simulink model "filter_mech_ell_noise"  (R2025b)
settings: Solver=VariableStepAuto  StartTime=0.0  StopTime=time(end)  RelTol=1e-3
values from neighbouring files (symbols this model uses):
  rpy = zeros(length(time),3)    [test_traj_gen_v2 1.m]    (also in test_traj_gen_v2.m)
  ST = 1/100    (= 0.01)    [test_traj_gen_v2 1.m]    (also in test_traj_gen_v2.m)
  vel_n = vel_n_f    [test_traj_gen_v2 1.m]    (also in test_traj_gen_v2.m)
undefined symbols (not defined in the file or in its folder): DiscIntNeverNeededParam
settings Model: Creator=Lorenzo  LastModifiedBy=roly2
settings RTWCC: GPUComputeCapability=3.5

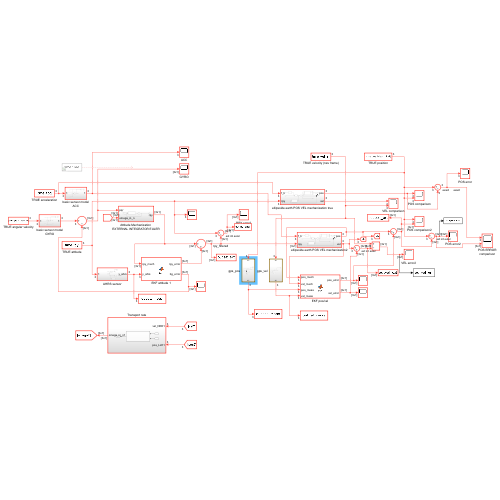
[thumbnail: Simulink's stored preview of the top-level diagram]
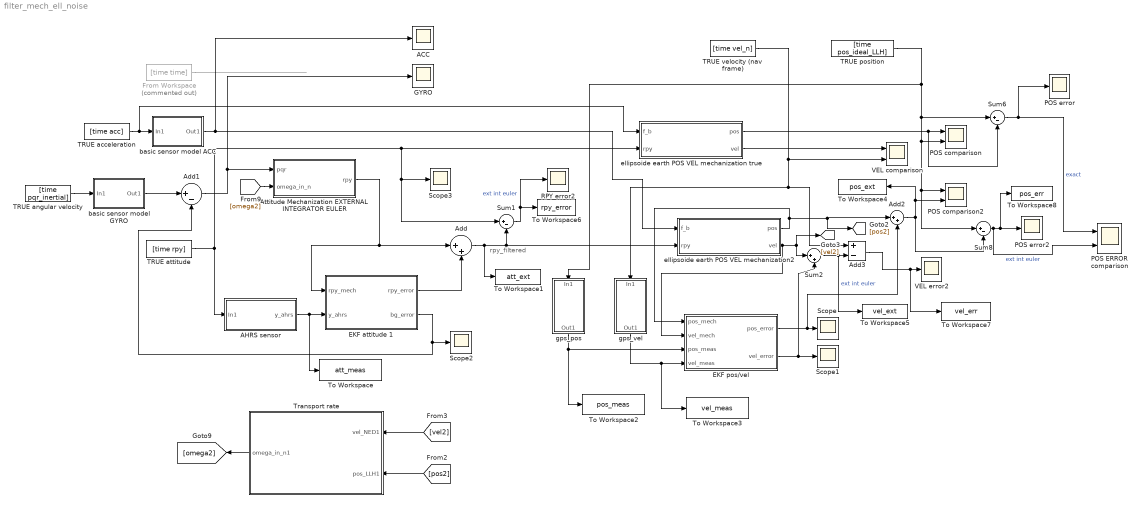
== system filter_mech_ell_noise ==
  note: rpy_filtered
  ACC : Scope
      settings: ActiveDisplayYMinimum=-11.440992557737301  ActiveDisplayYMaximum=2.4820081212415044  DataLoggingVariableName=ScopeData5
  AHRS sensor : Subsystem
  Add : Sum  Inputs=|++
  Add1 : Sum  Inputs=|+-
  Add2 : Sum  Inputs=|++
  Add3 : Sum  Inputs=+-
  Attitude Mechanization EXTERNAL INTEGRATOR EULER : Subsystem
  EKF attitude 1 : MATLAB Function  TreatAsAtomicUnit=on
  EKF pos/vel : MATLAB Function  TreatAsAtomicUnit=on
  From Workspace : FromWorkspace  Commented=on  VariableName=[time time]  SampleTime=ST
  GYRO : Scope
      settings: ActiveDisplayYMinimum=-0.0020882472519492545  ActiveDisplayYMaximum=0.00068115329120505431  DataLoggingVariableName=ScopeData12
  POS ERROR comparison : Scope  NumInputPorts=2
      settings: ActiveDisplayYMinimum=-0.463446142414341  ActiveDisplayYMaximum=0.1393650133582014  DataLoggingVariableName=ScopeData11
  POS comparison : Scope  NumInputPorts=2
      settings: ActiveDisplayYMinimum=19774.997277480568  ActiveDisplayYMaximum=20025.000302502158  DataLoggingVariableName=ScopeData2
  POS comparison2 : Scope  NumInputPorts=2
      settings: ActiveDisplayYMinimum=19774.812142318573  ActiveDisplayYMaximum=20025.022393794803
  POS error : Scope
      settings: ActiveDisplayYMinimum=-0.00026486838760320092  ActiveDisplayYMaximum=0.0023749580650473945  DataLoggingVariableName=ScopeData6
  POS error2 : Scope
      settings: ActiveDisplayYMinimum=-0.507273817207988  ActiveDisplayYMaximum=0.53432806462160443  DataLoggingVariableName=ScopeData8
  RPY error2 : Scope
      settings: ActiveDisplayYMinimum=-0.02159298222479724  ActiveDisplayYMaximum=0.026097778303773897
  Scope{,1..3} (4 alike) : Scope
      Scope settings: ActiveDisplayYMinimum=-5.2228791618423713  ActiveDisplayYMaximum=15.526847222191225
      Scope1 settings: ActiveDisplayYMinimum=0.5852793052063231  ActiveDisplayYMaximum=0.6306251008108662  DataLoggingVariableName=ScopeData9
      Scope2 settings: ActiveDisplayYMinimum=-0.0046074754298184107  ActiveDisplayYMaximum=0.0078155605686823729  DataLoggingVariableName=ScopeData16
      Scope3 settings: DataLoggingVariableName=ScopeData17
  Sum1 : Sum  Inputs=|+-
  Sum2 : Sum  Inputs=|++
  Sum6 : Sum  Inputs=|+-
  Sum8 : Sum  Inputs=|+-
  TRUE acceleration : FromWorkspace  VariableName=[time acc]  SampleTime=ST
  TRUE angular velocity : FromWorkspace  VariableName=[time pqr_inertial]  SampleTime=ST
  TRUE attitude : FromWorkspace  VariableName=[time rpy]  SampleTime=ST
  TRUE position : FromWorkspace  VariableName=[time pos_ideal_LLH]  SampleTime=ST
  TRUE velocity (nav frame) : FromWorkspace  VariableName=[time vel_n]  SampleTime=ST
  To Workspace : ToWorkspace  VariableName=att_meas  SaveFormat=Timeseries  SampleTime=-1
  To Workspace1 : ToWorkspace  VariableName=att_ext  SaveFormat=Timeseries  SampleTime=-1
  To Workspace2 : ToWorkspace  VariableName=pos_meas  SaveFormat=Timeseries  SampleTime=-1
  To Workspace3 : ToWorkspace  VariableName=vel_meas  SaveFormat=Timeseries  SampleTime=-1
  To Workspace4 : ToWorkspace  VariableName=pos_ext  SaveFormat=Timeseries  SampleTime=-1
  To Workspace5 : ToWorkspace  VariableName=vel_ext  SaveFormat=Timeseries  SampleTime=-1
  To Workspace6 : ToWorkspace  VariableName=rpy_error  SaveFormat=Timeseries  SampleTime=-1
  To Workspace7 : ToWorkspace  VariableName=vel_err  SaveFormat=Timeseries  SampleTime=-1
  To Workspace8 : ToWorkspace  VariableName=pos_err  SaveFormat=Timeseries  SampleTime=-1
  Transport rate : Subsystem
  VEL comparison : Scope  NumInputPorts=2
      settings: ActiveDisplayYMinimum=-163.77870347813263  ActiveDisplayYMaximum=201.30598005002113  DataLoggingVariableName=ScopeData3
  VEL error2 : Scope
      settings: ActiveDisplayYMinimum=-0.087937577094350031  ActiveDisplayYMaximum=0.084021536567730273  DataLoggingVariableName=ScopeData4
  basic sensor model ACC : Subsystem
  basic sensor model GYRO : Subsystem
  ellipsoide earth POS VEL mechanization true : Subsystem
  ellipsoide earth POS VEL mechanization2 : Subsystem
  gps_pos : Subsystem
  gps_vel : Subsystem
  wires:
  From Workspace/1 -> ?
  TRUE position/1 -> gps_pos/1(In1), POS comparison/2, Sum8/1, POS comparison2/1, Sum6/1
  TRUE velocity (nav frame)/1 -> Add3/1, gps_vel/1(In1), VEL comparison/2
  ellipsoide earth POS VEL mechanization true/1(pos) -> Sum6/2, POS comparison/1
  ellipsoide earth POS VEL mechanization true/2(vel) -> VEL comparison/1
  TRUE angular velocity/1 -> basic sensor model GYRO/1(In1)
  Attitude Mechanization EXTERNAL INTEGRATOR EULER/1(rpy) -> EKF attitude 1/1(rpy_mech), Add/1
  Sum1/1 -> To Workspace6/1, RPY error2/1  "ext int euler"
  TRUE attitude/1 -> AHRS sensor/1(In1), Scope3/1, Sum1/1, ellipsoide earth POS VEL mechanization true/2(rpy)
  Sum6/1 -> POS ERROR comparison/1, POS error/1  "exact"
  Sum8/1 -> POS ERROR comparison/2, To Workspace8/1, POS error2/1  "ext int euler"
  ellipsoide earth POS VEL mechanization2/1(pos) -> EKF pos/vel/1(pos_mech), [pos2], Add2/1
  basic sensor model ACC/1(Out1) -> ACC/1, ellipsoide earth POS VEL mechanization2/1(f_b)
  TRUE acceleration/1 -> ellipsoide earth POS VEL mechanization true/1(f_b), basic sensor model ACC/1(In1)
  basic sensor model GYRO/1(Out1) -> Add1/1
  ellipsoide earth POS VEL mechanization2/2(vel) -> EKF pos/vel/2(vel_mech), Sum2/1, [vel2]
  [omega2] -> Attitude Mechanization EXTERNAL INTEGRATOR EULER/2(omega_in_n)
  [vel2] -> Transport rate/1(vel_NED1)
  [pos2] -> Transport rate/2(pos_LLH1)
  Transport rate/1(omega_in_n1) -> [omega2]
  EKF attitude 1/2(bg_error) -> Scope2/1, Add1/2
  AHRS sensor/1(y_ahrs) -> To Workspace/1, EKF attitude 1/2(y_ahrs)
  EKF attitude 1/1(rpy_error) -> Add/2
  Add/1 -> To Workspace1/1, Sum1/2, ellipsoide earth POS VEL mechanization2/2(rpy)
  Add1/1 -> Attitude Mechanization EXTERNAL INTEGRATOR EULER/1(pqr), GYRO/1
  EKF pos/vel/2(vel_error) -> Scope1/1, Sum2/2
  EKF pos/vel/1(pos_error) -> Add2/2, Scope/1
  Add2/1 -> POS comparison2/2, To Workspace4/1, Sum8/2
  gps_pos/1(Out1) -> To Workspace2/1, EKF pos/vel/3(pos_meas)
  gps_vel/1(Out1) -> To Workspace3/1, EKF pos/vel/4(vel_meas)
  Sum2/1 -> To Workspace5/1, Add3/2  "ext int euler"
  Add3/1 -> To Workspace7/1, VEL error2/1

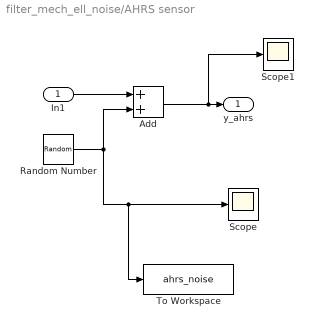
== system filter_mech_ell_noise/AHRS sensor ==
  In1 : Inport
  Add : Sum
  Random Number : RandomNumber  Mean=[0 0 0]  Variance=[0.0003 0.0003 0.0012]  Seed=[6 7 8]  SampleTime=ST
  Scope : Scope
      settings: ActiveDisplayYMinimum=-0.227023215913163  ActiveDisplayYMaximum=0.20537169700863794  DataLoggingVariableName=ScopeData13
  Scope1 : Scope
      settings: ActiveDisplayYMinimum=-0.036488467831931028  ActiveDisplayYMaximum=0.035623775404670058  DataLoggingVariableName=ScopeData14
  To Workspace : ToWorkspace  VariableName=ahrs_noise  SaveFormat=Timeseries  SampleTime=-1
  y_ahrs : Outport
  wires:
  Add/1 -> Scope1/1, y_ahrs/1
  In1/1 -> Add/1
  Random Number/1 -> To Workspace/1, Scope/1, Add/2

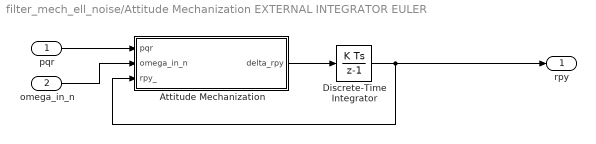
== system filter_mech_ell_noise/Attitude Mechanization EXTERNAL INTEGRATOR EULER ==
  pqr : Inport
  omega_in_n : Inport  Port=2
  Attitude Mechanization : MATLAB Function  TreatAsAtomicUnit=on
  Discrete-Time Integrator : DiscreteIntegrator  InitialCondition=rpy(1,:)'  SampleTime=ST  ICPrevOutput=DiscIntNeverNeededParam  ICPrevScaledInput=DiscIntNeverNeededParam
  rpy : Outport
  wires:
  Discrete-Time Integrator/1 -> rpy/1, Attitude Mechanization/3(rpy_)
  pqr/1 -> Attitude Mechanization/1(pqr)
  Attitude Mechanization/1(delta_rpy) -> Discrete-Time Integrator/1
  omega_in_n/1 -> Attitude Mechanization/2(omega_in_n)

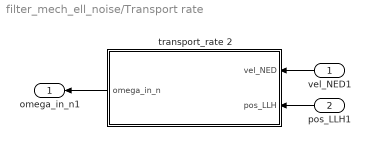
== system filter_mech_ell_noise/Transport rate ==
  vel_NED1 : Inport
  pos_LLH1 : Inport  Port=2
  transport_rate 2 : MATLAB Function  TreatAsAtomicUnit=on
  omega_in_n1 : Outport
  wires:
  pos_LLH1/1 -> transport_rate 2/2(pos_LLH)
  transport_rate 2/1(omega_in_n) -> omega_in_n1/1
  vel_NED1/1 -> transport_rate 2/1(vel_NED)

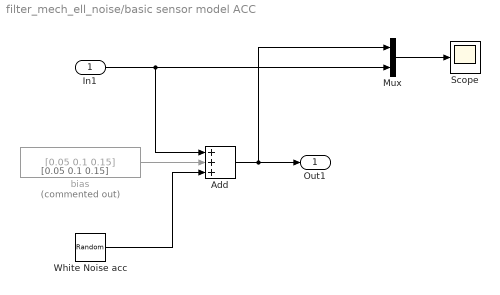
== system filter_mech_ell_noise/basic sensor model ACC ==
  note: [0.05 0.1 0.15]
  In1 : Inport
  Add : Sum  Inputs=+++
  Mux : Mux  Inputs=2
  Scope : Scope
      settings: ActiveDisplayYMinimum=-0.7520653966044506  ActiveDisplayYMaximum=0.75172983316287767
  White Noise acc : RandomNumber  DisableCoverage=on  Mean=[0 0 0 ]  Variance=[0.05 0.05 0.05].^2  Seed=[1 2 3]  SampleTime=ST
  bias : Constant  Commented=on  Value=[0.05 0.1 0.15]
  Out1 : Outport
  wires:
  In1/1 -> Mux/2, Add/1
  White Noise acc/1 -> Add/3
  bias/1 -> Add/2
  Mux/1 -> Scope/1
  Add/1 -> Mux/1, Out1/1

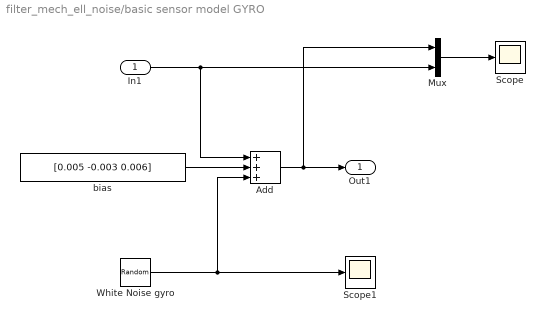
== system filter_mech_ell_noise/basic sensor model GYRO ==
  In1 : Inport
  Add : Sum  Inputs=+++
  Mux : Mux  Inputs=2
  Scope : Scope
      settings: ActiveDisplayYMinimum=-0.018561300716746276  ActiveDisplayYMaximum=0.027069948726320941  DataLoggingVariableName=ScopeData2
  Scope1 : Scope
      settings: ActiveDisplayYMinimum=-1  ActiveDisplayYMaximum=1  DataLoggingVariableName=ScopeData7
  White Noise gyro : RandomNumber  DisableCoverage=on  Mean=[0 0 0]  Variance=[0.003 0.003 0.003].^2  Seed=[4 5 6]  SampleTime=ST
  bias : Constant  Value=[0.005 -0.003 0.006]
  Out1 : Outport
  wires:
  White Noise gyro/1 -> Scope1/1, Add/3
  bias/1 -> Add/2
  Mux/1 -> Scope/1
  In1/1 -> Mux/2, Add/1
  Add/1 -> Mux/1, Out1/1

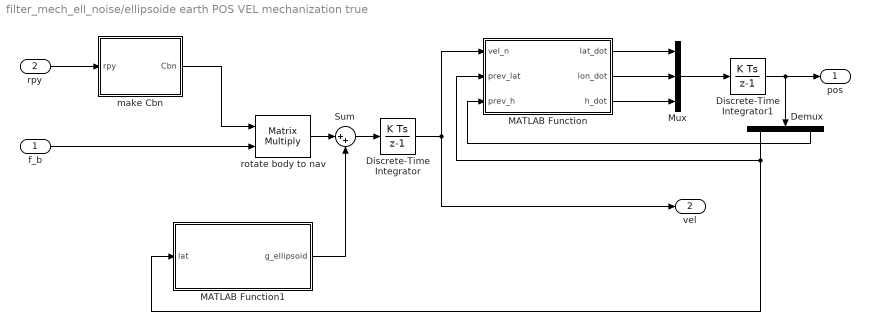
== system filter_mech_ell_noise/ellipsoide earth POS VEL mechanization true ==
  f_b : Inport
  rpy : Inport  Port=2
  Demux : Demux  Outputs=3
  Discrete-Time Integrator : DiscreteIntegrator  InitialCondition=vel_n(1,:)  SampleTime=-1  ICPrevOutput=DiscIntNeverNeededParam  ICPrevScaledInput=DiscIntNeverNeededParam
  Discrete-Time Integrator1 : DiscreteIntegrator  InitialCondition=[40.8522 * pi/180 ; 14.2681 * pi/180 ; 20000]  SampleTime=-1  ICPrevOutput=DiscIntNeverNeededParam  ICPrevScaledInput=DiscIntNeverNeededParam
  MATLAB Function : MATLAB Function  TreatAsAtomicUnit=on
  MATLAB Function1 : MATLAB Function  TreatAsAtomicUnit=on
  Mux : Mux  Inputs=3
  Sum : Sum  Inputs=|++
  make Cbn : MATLAB Function  TreatAsAtomicUnit=on
  rotate body to nav : Product  Multiplication=Matrix(*)
  pos : Outport
  vel : Outport  Port=2
  wires:
  rotate body to nav/1 -> Sum/1
  MATLAB Function1/1(g_ellipsoid) -> Sum/2
  Discrete-Time Integrator/1 -> MATLAB Function/1(vel_n), vel/1
  make Cbn/1(Cbn) -> rotate body to nav/1
  Sum/1 -> Discrete-Time Integrator/1
  f_b/1 -> rotate body to nav/2
  rpy/1 -> make Cbn/1(rpy)
  MATLAB Function/3(h_dot) -> Mux/3
  MATLAB Function/2(lon_dot) -> Mux/2
  MATLAB Function/1(lat_dot) -> Mux/1
  Mux/1 -> Discrete-Time Integrator1/1
  Discrete-Time Integrator1/1 -> pos/1, Demux/1
  Demux/1 -> MATLAB Function1/1(lat), MATLAB Function/2(prev_lat)
  Demux/3 -> MATLAB Function/3(prev_h)

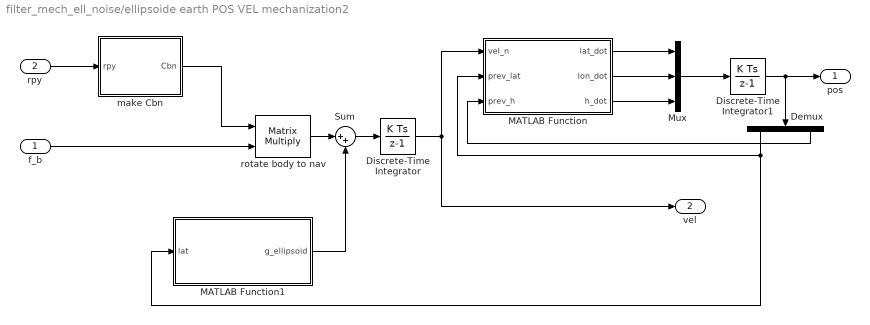
== system filter_mech_ell_noise/ellipsoide earth POS VEL mechanization2 ==
  f_b : Inport
  rpy : Inport  Port=2
  Demux : Demux  Outputs=3
  Discrete-Time Integrator : DiscreteIntegrator  InitialCondition=vel_n(1,:)  SampleTime=-1  ICPrevOutput=DiscIntNeverNeededParam  ICPrevScaledInput=DiscIntNeverNeededParam
  Discrete-Time Integrator1 : DiscreteIntegrator  InitialCondition=[40.8522 * pi/180 ; 14.2681 * pi/180 ; 20000]  SampleTime=-1  ICPrevOutput=DiscIntNeverNeededParam  ICPrevScaledInput=DiscIntNeverNeededParam
  MATLAB Function : MATLAB Function  TreatAsAtomicUnit=on
  MATLAB Function1 : MATLAB Function  TreatAsAtomicUnit=on
  Mux : Mux  Inputs=3
  Sum : Sum  Inputs=|++
  make Cbn : MATLAB Function  TreatAsAtomicUnit=on
  rotate body to nav : Product  Multiplication=Matrix(*)
  pos : Outport
  vel : Outport  Port=2
  wires:
  rotate body to nav/1 -> Sum/1
  Discrete-Time Integrator/1 -> MATLAB Function/1(vel_n), vel/1
  make Cbn/1(Cbn) -> rotate body to nav/1
  Sum/1 -> Discrete-Time Integrator/1
  f_b/1 -> rotate body to nav/2
  rpy/1 -> make Cbn/1(rpy)
  MATLAB Function/3(h_dot) -> Mux/3
  MATLAB Function/2(lon_dot) -> Mux/2
  MATLAB Function/1(lat_dot) -> Mux/1
  Mux/1 -> Discrete-Time Integrator1/1
  Discrete-Time Integrator1/1 -> pos/1, Demux/1
  Demux/3 -> MATLAB Function/3(prev_h)
  Demux/1 -> MATLAB Function1/1(lat), MATLAB Function/2(prev_lat)
  MATLAB Function1/1(g_ellipsoid) -> Sum/2

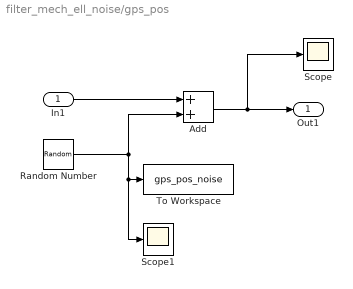
== system filter_mech_ell_noise/gps_pos ==
  In1 : Inport
  Add : Sum
  Random Number : RandomNumber  Mean=[0 0 0]  Variance=[1.5364e-13 1.5364e-13 12.25]  Seed=[3 4 5]  SampleTime=0.1
  Scope : Scope
      settings: ActiveDisplayYMinimum=20000.673472160557  ActiveDisplayYMaximum=20007.042526358724  DataLoggingVariableName=ScopeData15
  Scope1 : Scope
      settings: DataLoggingVariableName=ScopeData18
  To Workspace : ToWorkspace  VariableName=gps_pos_noise  SaveFormat=Timeseries  SampleTime=-1
  Out1 : Outport
  wires:
  Random Number/1 -> Scope1/1, To Workspace/1, Add/2
  Add/1 -> Scope/1, Out1/1
  In1/1 -> Add/1

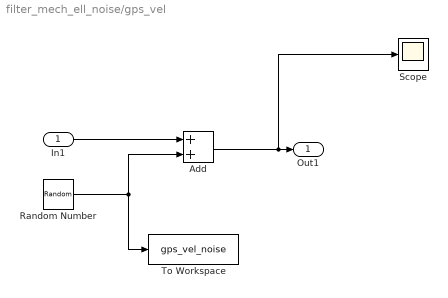
== system filter_mech_ell_noise/gps_vel ==
  In1 : Inport
  Add : Sum
  Random Number : RandomNumber  Mean=[0 0 0]  Variance=[0.0025 0.0025 0.0025]  Seed=[1 2 3]  SampleTime=0.1
  Scope : Scope
      settings: ActiveDisplayYMinimum=24.595394917727539  ActiveDisplayYMaximum=25.091783790953549  DataLoggingVariableName=ScopeData10
  To Workspace : ToWorkspace  VariableName=gps_vel_noise  SaveFormat=Timeseries  SampleTime=-1
  Out1 : Outport
  wires:
  In1/1 -> Add/1
  Add/1 -> Scope/1, Out1/1
  Random Number/1 -> To Workspace/1, Add/2

== matlab function filter_mech_ell_noise/ellipsoide earth POS VEL mechanization2/MATLAB Function1 ==
  data: lat input; g_ellipsoid output
function g_ellipsoid = gravity_compansation(lat)

g_wgs0 = 9.7803267714;
g_wgs1 = 0.00193185138639;

eps = 0.0818191908426;
eps2 = eps^2;

sin2phi = sin(lat)^2;
g = g_wgs0 * (1 + g_wgs1 * sin2phi) / sqrt(1 - eps2 * sin2phi);
g_ellipsoid = [0; 0; g];

== matlab function filter_mech_ell_noise/EKF pos//vel ==
  data: pos_mech input; pos_error output; vel_error output; vel_mech input; pos_meas input; vel_meas input; parameters parameter
function [pos_error, vel_error] = fcn(pos_mech, vel_mech, pos_meas, vel_meas, parameters)
    
    dt=parameters.dt_ekf;
    Q=parameters.Q_acc;
    R = parameters.R_gps;
   
    persistent x_hat P counter
    if isempty(x_hat)
        x_hat = zeros(6,1);   %Stato iniziale
        P=eye(6).*[0.01, 0.01, 0.01, 0.01, 0.01, 0.01];
        counter = 10;
    end
    
    %% Predizione
    [x_hat_pred, P_pred] = predict_EKF(x_hat, P, pos_mech, dt, Q);

    counter = counter + 1;

    if counter>= 10

        [x_hat , P] = correct_EKF(x_hat_pred , P_pred, pos_mech, vel_mech, pos_meas, vel_meas, R);
        counter = 0;

    else
        x_hat = x_hat_pred;
        P = P_pred;
    end

    pos_error = x_hat(1:3); 
    vel_error = x_hat(4:6);
    
end


function [x_hat_new , P_new] = predict_EKF(x_hat, P, pos_mech, dt, Q)

    phi = pos_mech(1);
    h = pos_mech(3);

    re = 6378137;
    eps = 0.0818191908426;
    eps2 = eps^2;

    sin2phi = sin(phi)^2;
    den = 1 - eps2 * sin2phi ; 

    R_N = re / (sqrt(den));
    R_M = R_N * (1 - eps2)/(den);

    Tr = zeros(3,3);

    Tr(1,1) = 1 / (R_M + h);
    Tr(2,2) = 1 / (R_N + h) / cos(phi);
    Tr(3,3) = -1;

    F = zeros(6,6);
    F(1:3,4:6) = Tr;
    G_cont = zeros(6,3);
    G_cont(4:6, 1:3) = eye(3);

    Q = eye(3) * Q;

    Fk = eye(6) + F * dt;
    Dk = G_cont * dt;
    
    % Predizione
    
    x_hat_new = Fk * x_hat;
    P_new = Fk*P*Fk' + Dk*Q*Dk';
end

function [x_hat_corr , P_corr]= correct_EKF(x_hat_pred , P_pred, pos_mech, vel_mech, pos_meas, vel_meas, R)
    z = [pos_meas - pos_mech;
        vel_meas - vel_mech];

    H = eye(6);

    h_exp = H * x_hat_pred;
    
    e = z - h_exp;     % Innovazione
   
    S = H*P_pred*H' + R;  % Covarianza dell'innovazione
    L = P_pred*H' / S;     % Guadagno Kalman
    
    x_hat_corr = x_hat_pred + L*e;
    I = eye(6);
    P_corr = (I-L*H)*P_pred*(I-L*H)'+L*R*L';  % Forma di Joseph
    
end

== matlab function filter_mech_ell_noise/EKF attitude 1 ==
  data: rpy_mech input; rpy_error output; bg_error output; y_ahrs input; parameters parameter
function [rpy_error, bg_error] = fcn(rpy_mech, y_ahrs, parameters)
    dt=parameters.dt_ekf;
    Q=parameters.Q;
    R = parameters.R_ahrs;
   
    persistent x_hat P bg_totale
    if isempty(x_hat)
        x_hat = zeros(6,1);   %Stato iniziale
        % x_hat(4:6) = [0.005; -0.003; 0.006];
        P=eye(6).*[0.01, 0.01, 0.01, 0.01, 0.01, 0.01];
        bg_totale = zeros(3,1);
    end
    
    %% Predizione
    [x_hat_pred, P_pred] = predict_EKF(x_hat, P, rpy_mech, dt, Q);
    
    [x_hat , P] = correct_EKF(x_hat_pred , P_pred, y_ahrs, rpy_mech, R);

    rpy_error = x_hat(1:3); % L'errore da sottrarre a rpy_mech
    bg_totale  = bg_totale + x_hat(4:6); % Il bias da sottrarre al giroscopio grezzo

    x_hat(4:6) = [0; 0; 0];

    bg_error = bg_totale;
    
end


function [x_hat_new , P_new] = predict_EKF(x_hat, P, rpy_mech, dt, Q)

    phi = rpy_mech(1); 
    theta = rpy_mech(2);
    % psi = rpy_mech(3);
    % 
    % % Calculate C_n_b
    % 
    % cph = cos(phi);   sph = sin(phi);
    % cth = cos(theta); sth = sin(theta);
    % cps = cos(psi);   sps = sin(psi);
    % 
    % C_b_n = [cth*cps,  sph*sth*cps - cph*sps,  cph*sth*cps + sph*sps;
    %      cth*sps,  sph*sth*sps + cph*cps,  cph*sth*sps - sph*cps;
    %      -sth,     sph*cth,                cph*cth];

    J = [1, sin(phi)*tan(theta), cos(phi)*tan(theta);
     0, cos(phi),            -sin(phi);
     0, sin(phi)/cos(theta), cos(phi)/cos(theta)];

    F = zeros(6,6);
    F(1:3, 4:6) = -J;
    G_cont = zeros(6,6);
    G_cont(1:3, 1:3) = -J;
    G_cont(4:6, 4:6) = eye(3);

    Q = diag([Q Q Q Q*1e-3 Q*1e-3 Q*1e-3]);

    Fk = eye(6) + F * dt;
    Dk = G_cont * dt;
    
    % Predizione
    
    x_hat_new = Fk * x_hat;
    P_new = Fk*P*Fk' + Dk*Q*Dk';
end

function [x_hat_corr , P_corr]= correct_EKF(x_hat_pred , P_pred, y_ahrs, rpy_mech, R)
    z = y_ahrs - rpy_mech;
    H = [eye(3), zeros(3,3)];

    h_exp = H * x_hat_pred;
    
    e = z - h_exp;     % Innovazione
   
    S = H*P_pred*H' + R;  % Covarianza dell'innovazione
    L = P_pred*H' / S;     % Guadagno Kalman
    
    x_hat_corr = x_hat_pred + L*e;
    I = eye(6);
    P_corr = (I-L*H)*P_pred*(I-L*H)'+L*R*L';  % Forma di Joseph
    
end

== matlab function filter_mech_ell_noise/ellipsoide earth POS VEL mechanization2/MATLAB Function ==
  data: vel_n input; lat_dot output; prev_lat input; prev_h input; lon_dot output; h_dot output
function [lat_dot, lon_dot, h_dot] = ellipsoid_mechanization(vel_n, prev_lat, prev_h)

vel_N = vel_n(1);
vel_E = vel_n(2);
vel_D = vel_n(3);

% Constants WGS-84

re = 6378137;
eps = 0.0818191908426;
eps2 = eps^2;

phi = prev_lat;
h = prev_h;

sin2phi = sin(phi)^2;
den = 1 - eps2 * sin2phi ; 

R_N = re / (sqrt(den));
R_M = R_N * (1 - eps2)/(den);

lat_dot = vel_N / (R_M + h);
lon_dot = vel_E / (R_N + h) / cos(phi) ;
h_dot = - vel_D;

end

== matlab function filter_mech_ell_noise/Attitude Mechanization EXTERNAL INTEGRATOR EULER/Attitude Mechanization ==
  data: pqr input; omega_in_n input; delta_rpy output; rpy_ input; ST parameter size=1
function delta_rpy = attitude_mech(pqr, omega_in_n, rpy_,ST)
%input:angular velocity at current timestep, latest estimation of attitude
%output> rpy and Cbn

phi = rpy_(1); 
theta = rpy_(2);
psi = rpy_(3);

% Calculate C_n_b

cph = cos(phi);   sph = sin(phi);
cth = cos(theta); sth = sin(theta);
cps = cos(psi);   sps = sin(psi);

C_b_n = [cth*cps,  sph*sth*cps - cph*sps,  cph*sth*cps + sph*sps;
         cth*sps,  sph*sth*sps + cph*cps,  cph*sth*sps - sph*cps;
         -sth,     sph*cth,                cph*cth];
C_n_b = C_b_n';

% Transport rate correction

pqr_corrected = pqr - C_n_b * omega_in_n;
%create Jacobian that transforms angular rates into rates of Euler
%angles
J = [1, sin(phi)*tan(theta), cos(phi)*tan(theta);
     0, cos(phi),            -sin(phi);
     0, sin(phi)/cos(theta), cos(phi)/cos(theta)];

%integrate
delta_rpy = J*pqr_corrected;

== matlab function filter_mech_ell_noise/ellipsoide earth POS VEL mechanization true/make Cbn ==
  data: rpy input; Cbn output
function Cbn = make_Cbn(rpy)
%compute Cbn
Cz=[cos(rpy(3))     sin(rpy(3))     0; ...
    -sin(rpy(3))    cos(rpy(3))     0; ...
    0               0               1];

Cy=[cos(rpy(2))     0               -sin(rpy(2)); ...
    0               1               0; ...
    sin(rpy(2))     0               cos(rpy(2))];

Cx=[1               0               0;...
    0               cos(rpy(1))     sin(rpy(1)); ...
    0               -sin(rpy(1))    cos(rpy(1))];

Cbn = (Cx*Cy*Cz)';

== matlab function filter_mech_ell_noise/ellipsoide earth POS VEL mechanization2/make Cbn ==
  data: rpy input; Cbn output
function Cbn = make_Cbn(rpy)
%compute Cbn
Cz=[cos(rpy(3))     sin(rpy(3))     0; ...
    -sin(rpy(3))    cos(rpy(3))     0; ...
    0               0               1];

Cy=[cos(rpy(2))     0               -sin(rpy(2)); ...
    0               1               0; ...
    sin(rpy(2))     0               cos(rpy(2))];

Cx=[1               0               0;...
    0               cos(rpy(1))     sin(rpy(1)); ...
    0               -sin(rpy(1))    cos(rpy(1))];

Cbn = (Cx*Cy*Cz)';

== matlab function filter_mech_ell_noise/ellipsoide earth POS VEL mechanization true/MATLAB Function ==
  data: vel_n input; lat_dot output; prev_lat input; prev_h input; lon_dot output; h_dot output
function [lat_dot, lon_dot, h_dot] = ellipsoid_mechanization(vel_n, prev_lat, prev_h)

vel_N = vel_n(1);
vel_E = vel_n(2);
vel_D = vel_n(3);

% Constants WGS-84

re = 6378137;
eps = 0.0818191908426;
eps2 = eps^2;

phi = prev_lat;
h = prev_h;

sin2phi = sin(phi)^2;
den = 1 - eps2 * sin2phi ; 

R_N = re / (sqrt(den));
R_M = R_N * (1 - eps2)/(den);

lat_dot = vel_N / (R_M + h);
lon_dot = vel_E / (R_N + h) / cos(phi) ;
h_dot = - vel_D;

end

== matlab function filter_mech_ell_noise/Transport rate/transport_rate 2 ==
  data: vel_NED input; omega_in_n output; pos_LLH input
function omega_in_n = transport_rate(vel_NED, pos_LLH)

v_N = vel_NED(1);
v_E = vel_NED(2);

phi = pos_LLH(1);
h = pos_LLH(3);

omega_E = 7.292115e-5; % Velocità di rotazione terrestre [rad/s]

re = 6378137;
eps = 0.0818191908426;
eps2 = eps^2;

sin2phi = sin(phi)^2;
den = 1 - eps2 * sin2phi;
R_N = re / (sqrt(den));
R_M = R_N * (1 - eps2) / den;

omega_ie_n = [omega_E * cos(phi) ; 0; -omega_E * sin(phi)];

omega_en_n = [  v_E / (R_N + h);
                -v_N / (R_M + h);
                -v_E * tan(phi) / (R_N + h)];

omega_in_n = omega_ie_n + omega_en_n;

end

== matlab function filter_mech_ell_noise/ellipsoide earth POS VEL mechanization true/MATLAB Function1 ==
  data: lat input; g_ellipsoid output
function g_ellipsoid = gravity_compansation(lat)

g_wgs0 = 9.7803267714;
g_wgs1 = 0.00193185138639;

eps = 0.0818191908426;
eps2 = eps^2;

sin2phi = sin(lat)^2;
g = g_wgs0 * (1 + g_wgs1 * sin2phi) / sqrt(1 - eps2 * sin2phi);
g_ellipsoid = [0; 0; g];
